simulink model "comms_test_cap_wc_xpc"  (Simulink 7.3)
settings: Solver=ode5  StartTime=0.0  StopTime=inf  FixedStep=0.0002  RelTol=1e-3
libraries: xpcutilitieslib x19, xpclib x6
settings Model: Creator=jporter  LastModifiedBy=jporter  BufferReuse=off
settings SolverCC: AutoInsertRateTranBlk=on
settings DataIOCC: LimitDataPoints=off  SaveOutput=off  SignalLogging=off  SaveTime=off
settings OptimizationCC: BlockReduction=off  OptimizeBlockIOStorage=off  BufferReuse=off  ExpressionFolding=off  LocalBlockOutputs=off  InitFltsAndDblsToZero=on
settings HardwareCC: ProdIntDivRoundTo=Zero  ProdEndianess=LittleEndian  ProdHWDeviceType=Generic->32-bit x86 compatible
settings RTWCC: SystemTargetFile=xpctarget.tlc  TemplateMakefile=xpc_default_tmf  Description=xPC Target  ProcessScript=xpctarget_make_rtw_hook  RTWCompilerOptimization=On
settings xpcTargetCC: TargetFcnLib=ansi_tfl_table_tmw.mat  TargetFunctionLibrary=ANSI_C  ParMdlRefBuildCompliant=off  PortableWordSizes=off  xPCisDownloadable=off

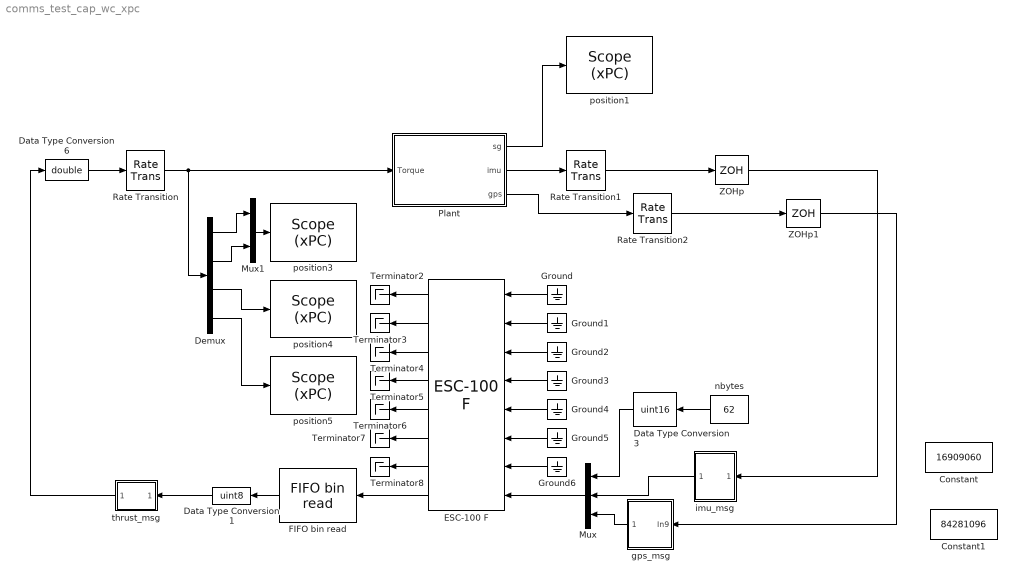
== system comms_test_cap_wc_xpc ==
  Constant : Constant  Value=16909060  OutDataTypeMode=uint32  OutDataType=sfix(16)  OutScaling=2^0  OutDataTypeStr=uint32  SampleTime=0.02
  Constant1 : Constant  Value=84281096  OutDataTypeMode=uint32  OutDataType=sfix(16)  OutScaling=2^0  OutDataTypeStr=uint32  SampleTime=0.02
  Data Type Conversion1 : DataTypeConversion  OutDataTypeMode=uint8  OutDataType=sfix(16)  OutScaling=2^0  OutDataTypeStr=uint8
  Data Type Conversion3 : DataTypeConversion  OutDataTypeMode=uint16  OutDataType=sfix(16)  OutScaling=2^0  OutDataTypeStr=uint16  ConvertRealWorld=Stored Integer (SI)
  Data Type Conversion6 : DataTypeConversion  OutDataTypeMode=double  OutDataType=sfix(16)  OutScaling=2^0  OutDataTypeStr=double
  Demux : Demux
  ESC-100 F : xpclib/RS232/Quatech/ESC-100/ESC-100 F  SystemSampleTime=-1  group=FIFO Setup  port=8  irqnum=10  slot=-1  baud1=57600  parity1=None  ndata1=8  nstop1=1  fifomode1=64 deep  rlevel1=half full  automode1=off  xmtfifosize1=1024  xmtdatatype1=count+16 bit uint  rcvfifosize1=1024  baud2=57600  parity2=None  ndata2=8  nstop2=1  fifomode2=64 deep  rlevel2=half full  automode2=off  xmtfifosize2=1024  xmtdatatype2=count+16 bit uint  rcvfifosize2=1024  baud3=57600  parity3=None  ndata3=8  nstop3=1  fifomode3=64 deep  rlevel3=half full  automode3=off  xmtfifosize3=1024  xmtdatatype3=count+16 bit uint  rcvfifosize3=1024  buad4=57600  parity4=None  ndata4=8  nstop4=1  fifomode4=64 deep  rlevel4=half full  automode4=off  xmtfifosize4=1024  xmtdatatype4=count+16 bit uint  rcvfifosize4=1024  baud5=57600  parity5=None  ndata5=8  nstop5=1  fifomode5=64 deep  rlevel5=half full  automode5=off  xmtfifosize5=1024  xmtdatatype5=count+16 bit uint  rcvfifosize5=1024  baud6=57600  parity6=None  ndata6=8  nstop6=1  fifomode6=64 deep  rlevel6=half full  automode6=off  xmtfifosize6=1024  xmtdatatype6=count+16 bit uint  rcvfifosize6=1024  baud7=57600  parity7=None  ndata7=8  nstop7=1  fifomode7=64 deep  rlevel7=half full  automode7=off  xmtfifosize7=1024  xmtdatatype7=count+16 bit uint  rcvfifosize7=1024  baud8=57600  parity8=None  ndata8=8  nstop8=1  fifomode8=64 deep  rlevel8=half full  automode8=off  xmtfifosize8=1024  xmtdatatype8=count+16 bit uint  rcvfifosize8=1024
  FIFO bin read : xpclib/RS232/FIFO bin read   header={char([147])}  lengths=[17]  hold=Zero output if no new data  enable=off  maxsize=17  outputtype=count+16 bit uint  sampletime=-1
  Ground{,1..6} (7 alike) : Ground
  Mux : Mux  Inputs=3
  Mux1 : Mux  Inputs=2
  Plant : Subsystem
  Rate Transition : RateTransition
  Rate Transition1 : RateTransition  OutPortSampleTimeOpt=Inherit  OutPortSampleTimeMultiple=2
  Rate Transition2 : RateTransition  OutPortSampleTimeOpt=Inherit  OutPortSampleTimeMultiple=2
  Terminator{2..8} (7 alike) : Terminator
  ZOHp : ZeroOrderHold  SampleTime=0.02
  ZOHp1 : ZeroOrderHold  SampleTime=0.1
  gps_msg : Subsystem
  imu_msg : Subsystem
  nbytes : Constant  Value=62  OutDataTypeMode=uint8  OutDataType=sfix(16)  OutScaling=2^0  OutDataTypeStr=uint8
  position1 : xpclib/Misc./Scope (xPC)   SystemSampleTime=-1  scopeno=1  scopetype=Target  autostart=on  viewmode=Graphical rolling  formatstr='%15.6f'  grid=on  ylimits=[-3,3]  nosamples=8000  noprepostsamples=0  interleave=100  triggermode=FreeRun  triggersignal=1  triggerlevel=0.0  triggerslope=Either  triggerscope=1  triggersample=0  filename=data.dat  mode=Lazy  writesize=512  autorestart=off
  position3 : xpclib/Misc./Scope (xPC)   SystemSampleTime=-1  scopeno=2  scopetype=Target  autostart=on  viewmode=Graphical rolling  formatstr='%15.6f'  grid=on  ylimits=[-3,3]  nosamples=8000  noprepostsamples=0  interleave=100  triggermode=FreeRun  triggersignal=1  triggerlevel=0.0  triggerslope=Either  triggerscope=1  triggersample=0  filename=data.dat  mode=Lazy  writesize=512  autorestart=off
  position4 : xpclib/Misc./Scope (xPC)   SystemSampleTime=-1  scopeno=3  scopetype=Target  autostart=on  viewmode=Graphical rolling  formatstr='%15.6f'  grid=on  ylimits=[-3,3]  nosamples=8000  noprepostsamples=0  interleave=100  triggermode=FreeRun  triggersignal=1  triggerlevel=0.0  triggerslope=Either  triggerscope=1  triggersample=0  filename=data.dat  mode=Lazy  writesize=512  autorestart=off
  position5 : xpclib/Misc./Scope (xPC)   SystemSampleTime=-1  scopeno=4  scopetype=Target  autostart=on  viewmode=Graphical rolling  formatstr='%15.6f'  grid=on  ylimits=[-3,3]  nosamples=8000  noprepostsamples=0  interleave=100  triggermode=FreeRun  triggersignal=1  triggerlevel=0.0  triggerslope=Either  triggerscope=1  triggersample=0  filename=data.dat  mode=Lazy  writesize=512  autorestart=off
  thrust_msg : Subsystem
  wires:
  Rate Transition/1 -> Plant/1(Torque), Demux/1
  ZOHp/1 -> imu_msg/1(In9)
  Data Type Conversion1/1 -> thrust_msg/1(In1)
  ESC-100 F/1 -> Terminator2/1
  ESC-100 F/2 -> Terminator3/1
  ESC-100 F/3 -> Terminator4/1
  ESC-100 F/4 -> Terminator5/1
  ESC-100 F/5 -> Terminator6/1
  ESC-100 F/6 -> Terminator7/1
  ESC-100 F/7 -> Terminator8/1
  Ground/1 -> ESC-100 F/1
  Ground1/1 -> ESC-100 F/2
  Ground2/1 -> ESC-100 F/3
  Ground3/1 -> ESC-100 F/4
  Ground4/1 -> ESC-100 F/5
  Ground5/1 -> ESC-100 F/6
  ESC-100 F/8 -> FIFO bin read/1
  FIFO bin read/1 -> Data Type Conversion1/1
  Rate Transition1/1 -> ZOHp/1
  Data Type Conversion6/1 -> Rate Transition/1
  thrust_msg/1(Out1) -> Data Type Conversion6/1
  Ground6/1 -> ESC-100 F/7
  Plant/2(imu) -> Rate Transition1/1
  Rate Transition2/1 -> ZOHp1/1
  Plant/3(gps) -> Rate Transition2/1
  Mux/1 -> ESC-100 F/8
  ZOHp1/1 -> gps_msg/1(In9)
  Plant/1(sg) -> position1/1
  nbytes/1 -> Data Type Conversion3/1
  imu_msg/1(Out1) -> Mux/2
  gps_msg/1(Out1) -> Mux/3
  Data Type Conversion3/1 -> Mux/1
  Mux1/1 -> position3/1
  Demux/1 -> Mux1/1
  Demux/2 -> Mux1/2
  Demux/3 -> position4/1
  Demux/4 -> position5/1

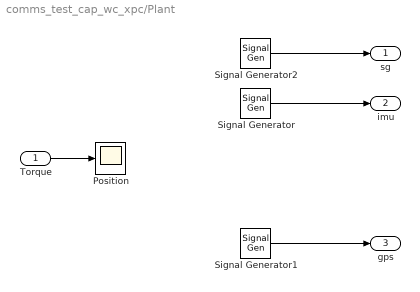
== system comms_test_cap_wc_xpc/Plant ==
  Torque : Inport
  Position : Scope
      settings: YMin=-20  YMax=20
  Signal Generator : SignalGenerator  Amplitude=ones(1,9)  Frequency=1/30
  Signal Generator1 : SignalGenerator  Amplitude=ones(1,6)  Frequency=1/30
  Signal Generator2 : SignalGenerator  Frequency=1/30
  sg : Outport
  imu : Outport  Port=2
  gps : Outport  Port=3
  wires:
  Signal Generator/1 -> imu/1
  Torque/1 -> Position/1
  Signal Generator1/1 -> gps/1
  Signal Generator2/1 -> sg/1

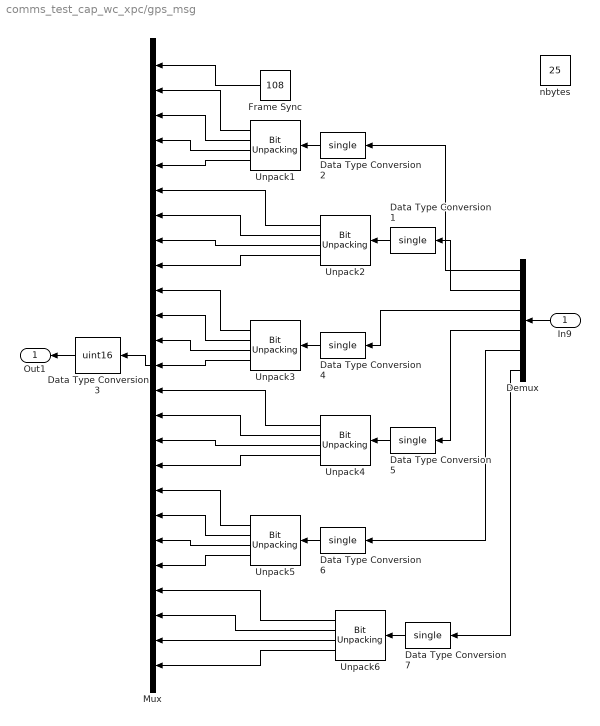
== system comms_test_cap_wc_xpc/gps_msg ==
  In9 : Inport
  Data Type Conversion{1..2,4..7} (6 alike) : DataTypeConversion  OutDataTypeMode=single  OutDataType=sfix(16)  OutScaling=2^0  OutDataTypeStr=single
  Data Type Conversion3 : DataTypeConversion  OutDataTypeMode=uint16  OutDataType=sfix(16)  OutScaling=2^0  OutDataTypeStr=uint16  ConvertRealWorld=Stored Integer (SI)
  Demux : Demux  Outputs=6
  Frame Sync : Constant  Value=108  OutDataTypeMode=uint8  OutDataType=sfix(16)  OutScaling=2^0  OutDataTypeStr=uint8
  Mux : Mux  Inputs=25
  Unpack{1..6} (6 alike) : xpcutilitieslib/Bit Unpacking   SignExtend=off  MaskBitPatterns={[0:7], [8:15], [16:23], [24:31]}  MaskPackDataType=single  MaskPackDataSize=[1]  MaskUnpackDataTypes={'uint8', 'uint8', 'uint8', 'uint8'}  MaskUnpackDataSizes={[1], [1], [1], [1]}
  nbytes : Constant  Value=25  OutDataTypeMode=uint8  OutDataType=sfix(16)  OutScaling=2^0  OutDataTypeStr=uint8
  Out1 : Outport
  wires:
  Mux/1 -> Data Type Conversion3/1
  Data Type Conversion2/1 -> Unpack1/1
  Data Type Conversion3/1 -> Out1/1
  Data Type Conversion1/1 -> Unpack2/1
  Data Type Conversion4/1 -> Unpack3/1
  Data Type Conversion5/1 -> Unpack4/1
  Data Type Conversion6/1 -> Unpack5/1
  Data Type Conversion7/1 -> Unpack6/1
  In9/1 -> Demux/1
  Demux/1 -> Data Type Conversion2/1
  Demux/2 -> Data Type Conversion1/1
  Demux/3 -> Data Type Conversion4/1
  Demux/4 -> Data Type Conversion5/1
  Demux/5 -> Data Type Conversion6/1
  Demux/6 -> Data Type Conversion7/1
  Frame Sync/1 -> Mux/1
  Unpack1/1 -> Mux/2
  Unpack1/2 -> Mux/3
  Unpack1/3 -> Mux/4
  Unpack1/4 -> Mux/5
  Unpack2/1 -> Mux/6
  Unpack2/2 -> Mux/7
  Unpack2/3 -> Mux/8
  Unpack2/4 -> Mux/9
  Unpack3/1 -> Mux/10
  Unpack3/2 -> Mux/11
  Unpack3/3 -> Mux/12
  Unpack3/4 -> Mux/13
  Unpack4/1 -> Mux/14
  Unpack4/2 -> Mux/15
  Unpack4/3 -> Mux/16
  Unpack4/4 -> Mux/17
  Unpack5/1 -> Mux/18
  Unpack5/2 -> Mux/19
  Unpack5/3 -> Mux/20
  Unpack5/4 -> Mux/21
  Unpack6/1 -> Mux/22
  Unpack6/2 -> Mux/23
  Unpack6/3 -> Mux/24
  Unpack6/4 -> Mux/25

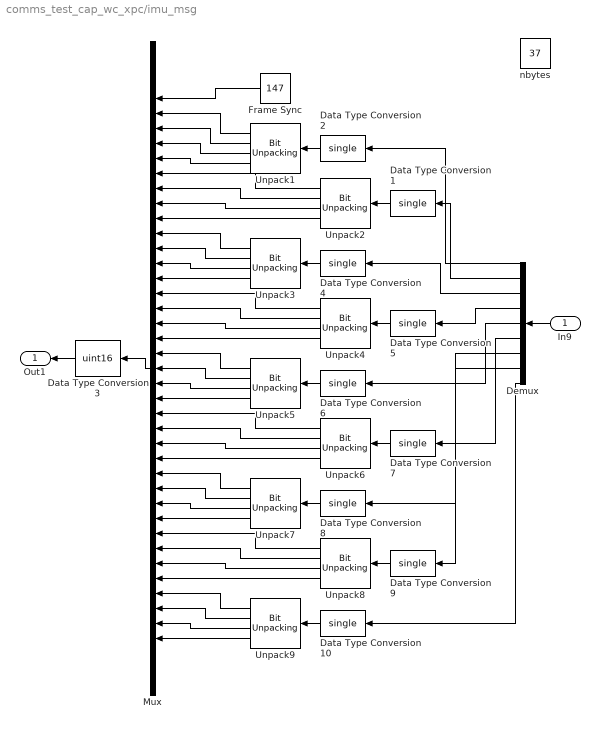
== system comms_test_cap_wc_xpc/imu_msg ==
  In9 : Inport
  Data Type Conversion{1..2,4..10} (9 alike) : DataTypeConversion  OutDataTypeMode=single  OutDataType=sfix(16)  OutScaling=2^0  OutDataTypeStr=single
  Data Type Conversion3 : DataTypeConversion  OutDataTypeMode=uint16  OutDataType=sfix(16)  OutScaling=2^0  OutDataTypeStr=uint16  ConvertRealWorld=Stored Integer (SI)
  Demux : Demux  Outputs=9
  Frame Sync : Constant  Value=147  OutDataTypeMode=uint8  OutDataType=sfix(16)  OutScaling=2^0  OutDataTypeStr=uint8
  Mux : Mux  Inputs=37
  Unpack{1..9} (9 alike) : xpcutilitieslib/Bit Unpacking   SignExtend=off  MaskBitPatterns={[0:7], [8:15], [16:23], [24:31]}  MaskPackDataType=single  MaskPackDataSize=[1]  MaskUnpackDataTypes={'uint8', 'uint8', 'uint8', 'uint8'}  MaskUnpackDataSizes={[1], [1], [1], [1]}
  nbytes : Constant  Value=37  OutDataTypeMode=uint8  OutDataType=sfix(16)  OutScaling=2^0  OutDataTypeStr=uint8
  Out1 : Outport
  wires:
  Mux/1 -> Data Type Conversion3/1
  Data Type Conversion2/1 -> Unpack1/1
  Data Type Conversion3/1 -> Out1/1
  Data Type Conversion1/1 -> Unpack2/1
  Data Type Conversion4/1 -> Unpack3/1
  Data Type Conversion5/1 -> Unpack4/1
  Data Type Conversion6/1 -> Unpack5/1
  Data Type Conversion7/1 -> Unpack6/1
  Data Type Conversion8/1 -> Unpack7/1
  Data Type Conversion9/1 -> Unpack8/1
  Data Type Conversion10/1 -> Unpack9/1
  In9/1 -> Demux/1
  Demux/1 -> Data Type Conversion2/1
  Demux/2 -> Data Type Conversion1/1
  Demux/3 -> Data Type Conversion4/1
  Demux/4 -> Data Type Conversion5/1
  Demux/5 -> Data Type Conversion6/1
  Demux/6 -> Data Type Conversion7/1
  Demux/7 -> Data Type Conversion8/1
  Demux/8 -> Data Type Conversion9/1
  Demux/9 -> Data Type Conversion10/1
  Frame Sync/1 -> Mux/1
  Unpack1/1 -> Mux/2
  Unpack1/2 -> Mux/3
  Unpack1/3 -> Mux/4
  Unpack1/4 -> Mux/5
  Unpack2/1 -> Mux/6
  Unpack2/2 -> Mux/7
  Unpack2/3 -> Mux/8
  Unpack2/4 -> Mux/9
  Unpack3/1 -> Mux/10
  Unpack3/2 -> Mux/11
  Unpack3/3 -> Mux/12
  Unpack3/4 -> Mux/13
  Unpack4/1 -> Mux/14
  Unpack4/2 -> Mux/15
  Unpack4/3 -> Mux/16
  Unpack4/4 -> Mux/17
  Unpack5/1 -> Mux/18
  Unpack5/2 -> Mux/19
  Unpack5/3 -> Mux/20
  Unpack5/4 -> Mux/21
  Unpack6/1 -> Mux/22
  Unpack6/2 -> Mux/23
  Unpack6/3 -> Mux/24
  Unpack6/4 -> Mux/25
  Unpack7/1 -> Mux/26
  Unpack7/2 -> Mux/27
  Unpack7/3 -> Mux/28
  Unpack7/4 -> Mux/29
  Unpack8/1 -> Mux/30
  Unpack8/2 -> Mux/31
  Unpack8/3 -> Mux/32
  Unpack8/4 -> Mux/33
  Unpack9/1 -> Mux/34
  Unpack9/2 -> Mux/35
  Unpack9/3 -> Mux/36
  Unpack9/4 -> Mux/37

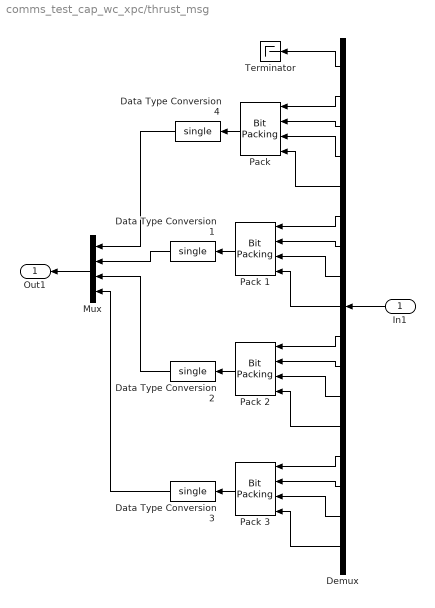
== system comms_test_cap_wc_xpc/thrust_msg ==
  In1 : Inport
  Data Type Conversion{1..4} (4 alike) : DataTypeConversion  OutDataTypeMode=single  OutDataType=sfix(16)  OutScaling=2^0  OutDataTypeStr=single
  Demux : Demux  Outputs=17
  Mux : Mux
  Pack {,1..3} (4 alike) : xpcutilitieslib/Bit Packing   MaskBitPatterns={[0:7], [8:15], [16:23], [24:31]}  MaskPackDataType=single  MaskPackDataSize=[1]
  Terminator : Terminator
  Out1 : Outport
  wires:
  Demux/1 -> Terminator/1
  "Pack "/1 -> Data Type Conversion4/1
  Demux/2 -> "Pack "/1
  Demux/3 -> "Pack "/2
  Demux/4 -> "Pack "/3
  Demux/5 -> "Pack "/4
  In1/1 -> Demux/1
  Pack 1/1 -> Data Type Conversion1/1
  Demux/6 -> Pack 1/1
  Demux/7 -> Pack 1/2
  Demux/8 -> Pack 1/3
  Demux/9 -> Pack 1/4
  Pack 2/1 -> Data Type Conversion2/1
  Demux/10 -> Pack 2/1
  Demux/11 -> Pack 2/2
  Demux/12 -> Pack 2/3
  Demux/13 -> Pack 2/4
  Pack 3/1 -> Data Type Conversion3/1
  Demux/14 -> Pack 3/1
  Demux/15 -> Pack 3/2
  Demux/16 -> Pack 3/3
  Demux/17 -> Pack 3/4
  Data Type Conversion4/1 -> Mux/1
  Mux/1 -> Out1/1
  Data Type Conversion1/1 -> Mux/2
  Data Type Conversion2/1 -> Mux/3
  Data Type Conversion3/1 -> Mux/4
